simulink model "Ej_1b_1c_1d_simulink_2016"  (R2016a)
settings: Solver=VariableStepAuto  SolverMode=SingleTasking  StartTime=0.0  StopTime=10.0  RelTol=1e-3
values from neighbouring files (symbols this model uses):
  G = 6 / (s+1)    [Ej_1a.m]    (also in Ej_1b.m = 10 / ((s+1)*(s+2)); Ej_1c.m = 6 / (s*(s+2)); Ej_1d.m = (s+1) / (s^2 + 2*s + 1))
  H = 1    [Ej_1a.m]    (also in Ej_1b.m = 1 / (s+3); Ej_1c.m = 5 / (s+2); Ej_1d.m = 4 / (s+4))
settings Model: Creator=saldi  LastModifiedBy=saldi
settings DataIOCC: ReturnWorkspaceOutputs=on
settings DebuggingCC: UnconnectedInputMsg=none  UnconnectedOutputMsg=none  UnconnectedLineMsg=none  SFUnexpectedBacktrackingDiag=error  SFNoUnconditionalDefaultTransitionDiag=error
settings ModelReferenceCC: EnableRefExpFcnMdlSchedulingChecks=off
settings SFSimCC: SimUseLocalCustomCode=on
settings RTWCC: Description=Generic Real-Time Target  RTWUseLocalCustomCode=on
settings GRTTargetCC: TargetLangStandard=C99 (ISO)
settings ConfigComp: CovMetricSettings=dwe  CovSaveCumulativeToWorkspaceVar=off  CovSaveSingleToWorkspaceVar=off  CovExternalEMLEnable=on

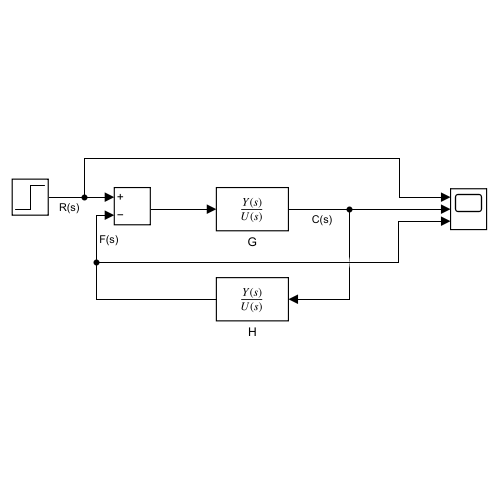
[thumbnail: Simulink's stored preview of the top-level diagram]
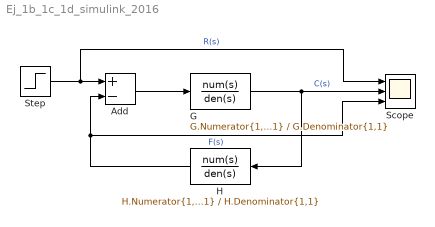
== system Ej_1b_1c_1d_simulink_2016 ==
  Add : Sum  Inputs=+-
  G : TransferFcn  Numerator=G.Numerator{1,1}  Denominator=G.Denominator{1,1}
  H : TransferFcn  Numerator=H.Numerator{1,1}  Denominator=H.Denominator{1,1}
  Scope : Scope  NumInputPorts=3
  Step : Step  SampleTime=0
  wires:
  G/1 -> H/1, Scope/2  "C(s)"
  Add/1 -> G/1
  Step/1 -> Scope/1, Add/1  "R(s)"
  H/1 -> Add/2, Scope/3  "F(s)"
